simulink model "model"  (R2020b)
settings: Solver=VariableStepAuto  StartTime=0.0  StopTime=1  RelTol=1e-3
settings Model: Creator=Lenovo  LastModifiedBy=Lenovo

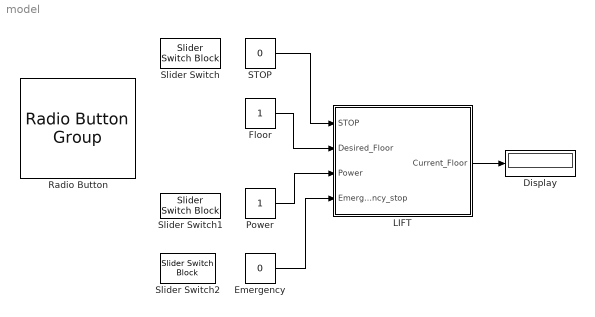
== system model ==
  Display : Display
  Emergency : Constant  Value=0
  Floor : Constant
  "LIFT " : Stateflow chart  TreatAsAtomicUnit=on
  Power : Constant
  Radio Button : RadioButtonGroup  LabelPosition=Bottom  SelectedLabel="First  Floor"  ButtonGroupName=Group
      settings: Values={{'First  Floor', 'Second Floor', 'Third Floor', 'Fourth Floor', 'Fifth Floor'}, [1 2 3 4 5]}
  STOP : Constant  Value=0
  Slider Switch : SliderSwitchBlock
      settings: Values={{'Off', 'On'}, [0 1]}
  Slider Switch1 : SliderSwitchBlock
      settings: Values={{'Off', 'On'}, [0 1]}
  Slider Switch2 : SliderSwitchBlock
      settings: Values={{'Off', 'On'}, [0 1]}
  wires:
  Power/1 -> "LIFT "/3(Power)
  Emergency/1 -> "LIFT "/4(Emergency_stop)
  Floor/1 -> "LIFT "/2(Desired_Floor)
  "LIFT "/1(Current_Floor) -> Display/1
  STOP/1 -> "LIFT "/1(STOP)

== stateflow chart model/LIFT  ==
  state Lift [parallel]
    settings: executionOrder=1
    (history)
    state Power
    state NORMAL
      state Loop1 [parallel]
        settings: executionOrder=1
        (history)
        state Emer
          en:
        state Loop2
        (default) -> Emer
        Emer -> Loop2 : [Emergency_stop==0]{send(No_emg,Emergency)}
        Loop2 -> Emer : [Emergency_stop==1]{send(Emg,Emergency)}
      state Emergency [parallel]
        settings: executionOrder=2
        (history)
        state Emg_off
          en:
        state Emg_On
          en:
          disp 'EMERGENCY STOP AND ALARM ARE ON';
        (default) -> Emg_off
        Emg_off -> Emg_On : Emg
        Emg_On -> Emg_off : No_emg{disp 'EMERGENCY STOP AND ALARM ARE OFF'}
    (default) -> Power
    Power -> NORMAL : [Power==1]{disp 'Power On'}
    NORMAL -> Power : [Power==0]{disp 'Power Off'}
  data: i local; STOP input; Current_Floor output; Desired_Floor input; Power input; Emergency_stop input
  events: Emg local FUNCTION_CALL_EVENT; No_emg local FUNCTION_CALL_EVENT; Off local FUNCTION_CALL_EVENT; On local FUNCTION_CALL_EVENT
